simulink model "tarea"  (R2022a)
settings: Solver=ode4  StartTime=0.0  StopTime=50  FixedStep=0.001  RelTol=1e-3
settings Model: Creator=Ari  LastModifiedBy=Ari

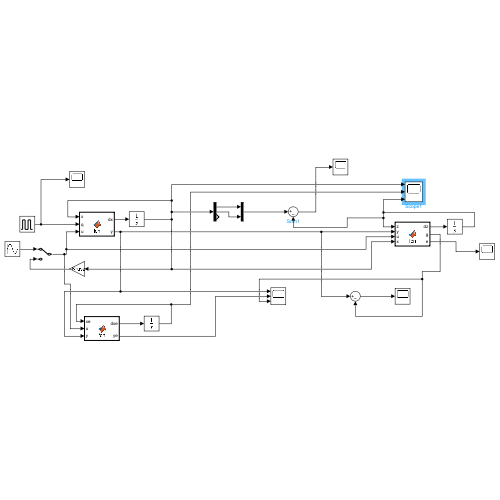
[thumbnail: Simulink's stored preview of the top-level diagram]
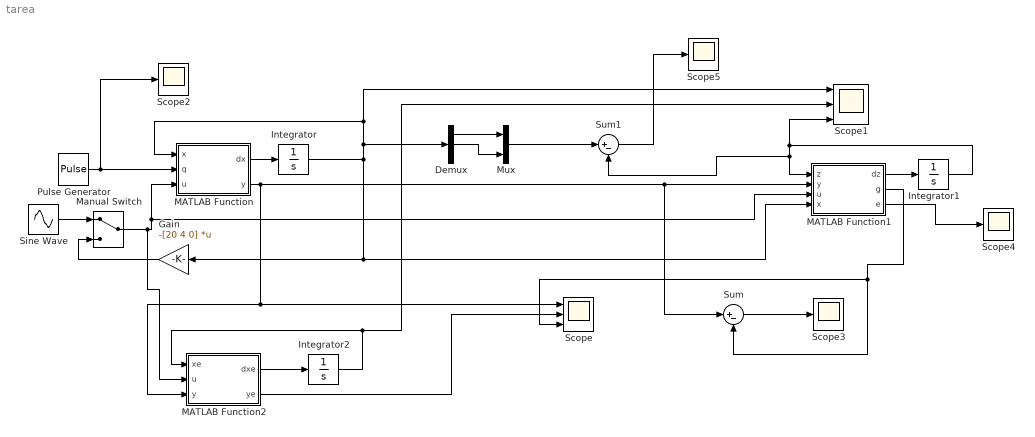
== system tarea ==
  Demux : Demux  Outputs=3
  Gain : Gain  Gain=-[20 4 0]  Multiplication=Matrix(K*u) (u vector)
  Integrator : Integrator  InitialCondition=[1;1;1]
  Integrator1 : Integrator  InitialCondition=[1;1]
  Integrator2 : Integrator  InitialCondition=[1;1;1]
  MATLAB Function : MATLAB Function  TreatAsAtomicUnit=on
  MATLAB Function1 : MATLAB Function  TreatAsAtomicUnit=on
  MATLAB Function2 : MATLAB Function  TreatAsAtomicUnit=on
  Manual Switch : ManualSwitch
  Mux : Mux  Inputs=2
  Pulse Generator : DiscretePulseGenerator  PulseType=Time based  Amplitude=0  PulseWidth=40
  Scope : Scope  NumInputPorts=3
  Scope1 : Scope  NumInputPorts=3
  Scope{2..5} (4 alike) : Scope
  Sine Wave : Sin  SampleTime=0
  Sum : Sum  Inputs=|+-
  Sum1 : Sum  Inputs=|+-
  wires:
  MATLAB Function/1(dx) -> Integrator/1
  Integrator/1 -> Gain/1, MATLAB Function1/4(x), Demux/1, MATLAB Function/1(x), Scope1/1
  MATLAB Function/2(y) -> MATLAB Function2/3(y), Scope/1, Sum/1, MATLAB Function1/2(y)
  MATLAB Function1/1(dz) -> Integrator1/1
  Integrator1/1 -> Sum1/2, MATLAB Function1/1(z), Scope1/3
  MATLAB Function2/1(dxe) -> Integrator2/1
  Integrator2/1 -> Scope1/2, MATLAB Function2/1(xe)
  MATLAB Function2/2(ye) -> Scope/2
  MATLAB Function1/2(g) -> Sum/2, Scope/3
  Pulse Generator/1 -> Scope2/1, MATLAB Function/2(q)
  Sum/1 -> Scope3/1
  MATLAB Function1/3(e) -> Scope4/1
  Sine Wave/1 -> Manual Switch/1
  Gain/1 -> Manual Switch/2
  Manual Switch/1 -> MATLAB Function2/2(u), MATLAB Function1/3(u), MATLAB Function/3(u)
  Demux/1 -> Mux/1
  Demux/2 -> Mux/2
  Mux/1 -> Sum1/1
  Sum1/1 -> Scope5/1

== matlab function tarea/MATLAB Function1 ==
  data: z input; dz output; g output; y input; u input; x input; e output
function [dz,g,e] = fcn(z,y,u,x)
A=[2 1 0;0 -3 0;-1 0 -1];
B=[0 1 0]';
C=[0 1 0;0 0 1];
D=[1 0;-2 0;0 2];
A0=A+D*C;
P=[1 0 0;0 1 0];
Pi=[1 0;0 1;0 0];
F=P*A0*Pi;
%M=C*Pi;
M=[0 1;0 0];
G=P*B;
dz=F*z+G*u-E*y;
g=M*z;
e=z-P*x;

== matlab function tarea/MATLAB Function ==
  data: x input; q input; u input; dx output; y output
function [dx,y] = fcn(x,q,u)
A=[2 1 0;0 -3 0;-1 0 -1];
B=[0 1 0]';
C=[0 1 0;0 0 1];
L=[0 0 1]';
y=C*x;
dx=A*x+B*u+L*q;

== matlab function tarea/MATLAB Function2 ==
  data: xe input; u input; y input; dxe output; ye output
function [dxe,ye] = fcn(xe,u,y)
A=[2 1 0;0 -3 0;-1 0 -1];
B=[0 1 0]';
C=[0 1 0;0 0 1];
D=[1 0;1 0;0 2];
ye=C*xe;
dxe=A*xe+B*u+D*(y-ye);
